simulink model "HDLQAMDemod"  (R2024a)
settings: Solver=FixedStepDiscrete  StartTime=0.0  StopTime=stopTime  RelTol=1e-3
undefined symbols (not defined in the file or in its folder): CONST
libraries: dspsrcs4 x3, HDL_ieee_8021513 x2, whdlutilities x1
settings Model: DataTypeOverride=Off  Creator=cotti  LastModifiedBy=cotti
settings OptimizationCC: BlockReduction=off  ConditionallyExecuteInputs=off  DefaultParameterBehavior=Inlined  InheritOutputTypeSmallerThanSingle=on
settings DebuggingCC: AlgebraicLoopMsg=error  ArtificialAlgebraicLoopMsg=error  SingleTaskRateTransMsg=error  UnconnectedInputMsg=warning  UnconnectedOutputMsg=warning  UnconnectedLineMsg=warning
settings HardwareCC: ProdBitPerPointer=32  ProdBitPerSizeT=32  ProdBitPerPtrDiffT=32  ProdLargestAtomicFloat=None  ProdIntDivRoundTo=Undefined  ProdEndianess=Unspecified  ProdWordSize=32  ProdHWDeviceType=ASIC/FPGA->ASIC/FPGA  TargetBitPerLong=64  TargetBitPerPointer=64  TargetBitPerSizeT=64  TargetBitPerPtrDiffT=64  TargetLongLongMode=on  TargetIntDivRoundTo=Zero  TargetEndianess=LittleEndian  TargetWordSize=64  TargetHWDeviceType=Custom Processor->MATLAB Host Computer  ProdEqTarget=off

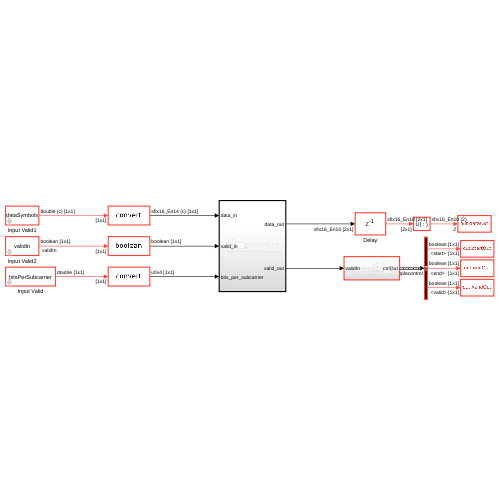
[thumbnail: Simulink's stored preview of the top-level diagram]
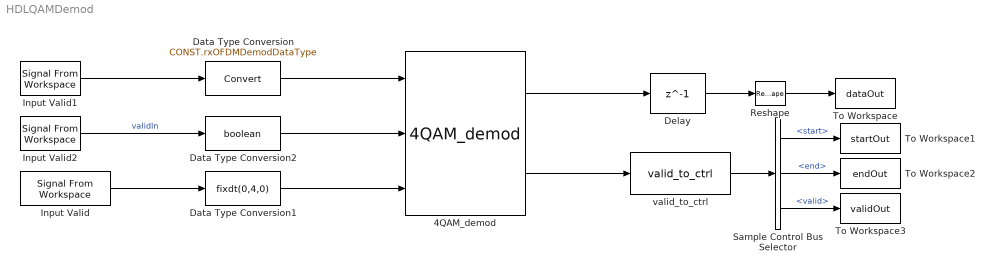
== system HDLQAMDemod ==
  4QAM_demod : HDL_ieee_8021513/4QAM_demod  SystemSampleTime=-1  VariantActivationTime=update diagram  AllowFlexibleInterface=on  Latency=0  AutoFrameSizeCalculation=off
      settings: SourceProductName=HDL IEEE 8021513
  Data Type Conversion : DataTypeConversion  OutDataTypeStr=CONST.rxOFDMDemodDataType  SaturateOnIntegerOverflow=off  RndMeth=Floor
  Data Type Conversion1 : DataTypeConversion  OutDataTypeStr=fixdt(0,4,0)  SaturateOnIntegerOverflow=off  RndMeth=Floor
  Data Type Conversion2 : DataTypeConversion  OutDataTypeStr=boolean  SaturateOnIntegerOverflow=off  RndMeth=Floor
  Delay : Delay  DelayLength=1  InitialCondition=0  UseCircularBuffer=on
  Input Valid : dspsrcs4/Signal From Workspace  X=bitsPerSubcarrier  Ts=1/CONST.fs  nsamps=1  OutputAfterFinalValue=Setting to zero  ignoreOrWarnInputAndFrameLengths=off  OutputFrames=off
  Input Valid1 : dspsrcs4/Signal From Workspace  X=dataSymbols  Ts=1/CONST.fs  nsamps=1  OutputAfterFinalValue=Setting to zero  ignoreOrWarnInputAndFrameLengths=off  OutputFrames=off
  Input Valid2 : dspsrcs4/Signal From Workspace  X=validIn  Ts=1/CONST.fs  nsamps=1  OutputAfterFinalValue=Setting to zero  ignoreOrWarnInputAndFrameLengths=off  OutputFrames=off
  Reshape : Reshape
  Sample Control Bus Selector : whdlutilities/Sample Control Bus Selector  OutputSignals=start,end,valid
  To Workspace : ToWorkspace  VariableName=dataOut  SampleTime=1/CONST.fs
      settings: Save2DSignal=2-D array (concatenate along first dimension)
  To Workspace1 : ToWorkspace  VariableName=startOut  SampleTime=1/CONST.fs
      settings: Save2DSignal=2-D array (concatenate along first dimension)
  To Workspace2 : ToWorkspace  VariableName=endOut  SampleTime=1/CONST.fs
      settings: Save2DSignal=2-D array (concatenate along first dimension)
  To Workspace3 : ToWorkspace  VariableName=validOut  SampleTime=1/CONST.fs
      settings: Save2DSignal=2-D array (concatenate along first dimension)
  valid_to_ctrl : HDL_ieee_8021513/valid_to_ctrl  SystemSampleTime=-1  VariantActivationTime=update diagram  AllowFlexibleInterface=on  Latency=0  AutoFrameSizeCalculation=off
      settings: SourceProductName=HDL IEEE 8021513
  wires:
  Sample Control Bus Selector/2 -> To Workspace2/1  "<end>"
  Input Valid/1 -> Data Type Conversion1/1
  4QAM_demod/2 -> valid_to_ctrl/1
  Input Valid2/1 -> Data Type Conversion2/1  "validIn"
  Sample Control Bus Selector/3 -> To Workspace3/1  "<valid>"
  Input Valid1/1 -> Data Type Conversion/1
  Data Type Conversion/1 -> 4QAM_demod/1
  valid_to_ctrl/1 -> Sample Control Bus Selector/1
  Sample Control Bus Selector/1 -> To Workspace1/1  "<start>"
  Delay/1 -> Reshape/1
  Data Type Conversion1/1 -> 4QAM_demod/3
  Data Type Conversion2/1 -> 4QAM_demod/2
  Reshape/1 -> To Workspace/1
  4QAM_demod/1 -> Delay/1
